simulink model "HW6_46"  (R2017a)
settings: Solver=VariableStepAuto  StartTime=0.0  StopTime=30  RelTol=1e-3
settings Model: Creator=USER  LastModifiedBy=dell

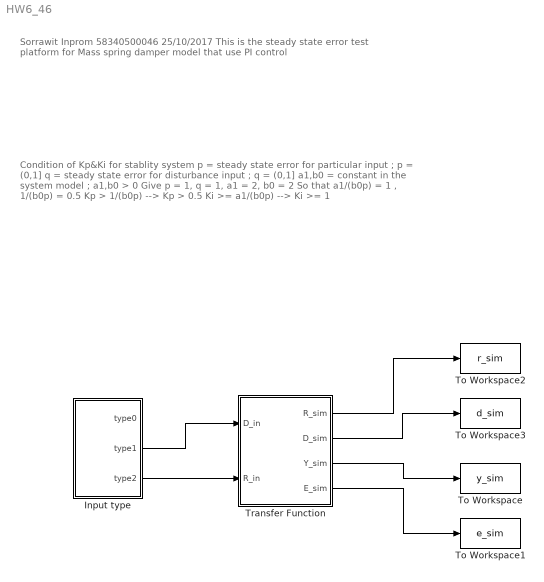
== system HW6_46 ==
  note: Sorrawit Inprom 58340500046
      | 25/10/2017
      |
      | This is the steady state error test platform
      | for Mass spring damper model that use PI control
  note: Condition of Kp&Ki for stablity system
      |
      | p = steady state error for particular input ; p = (0,1]
      | q = steady state error for disturbance input ; q = (0,1]
      | a1,b0 = constant in the system model ; a1,b0 > 0
      |
      | Give p = 1, q = 1, a1 = 2, b0 = 2
      |
      | So that a1/(b0p) = 1 , 1/(b0p) = 0.5
      |
      | Kp > 1/(b0p) --> Kp > 0.5
      | Ki >= a1/(b0p) --> Ki >= 1
  Input type : Subsystem
  To Workspace : ToWorkspace  VariableName=y_sim  SaveFormat=Timeseries  SampleTime=-1
  To Workspace1 : ToWorkspace  VariableName=e_sim  SaveFormat=Timeseries  SampleTime=-1
  To Workspace2 : ToWorkspace  VariableName=r_sim  SaveFormat=Timeseries  SampleTime=-1
  To Workspace3 : ToWorkspace  VariableName=d_sim  SaveFormat=Timeseries  SampleTime=-1
  Transfer Function : Subsystem  mask{a1=2, b0=2, Kp=1, Ki=1}
  wires:
  Transfer Function/1(R_sim) -> To Workspace2/1
  Transfer Function/2(D_sim) -> To Workspace3/1
  Transfer Function/3(Y_sim) -> To Workspace/1
  Transfer Function/4(E_sim) -> To Workspace1/1
  Input type/3(type2) -> Transfer Function/2(R_in)
  Input type/2(type1) -> Transfer Function/1(D_in)

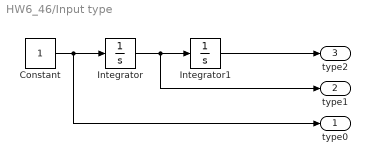
== system HW6_46/Input type ==
  Constant : Constant
  Integrator : Integrator
  Integrator1 : Integrator
  type0 : Outport
  type1 : Outport  Port=2
  type2 : Outport  Port=3
  wires:
  Integrator/1 -> type1/1, Integrator1/1
  Constant/1 -> type0/1, Integrator/1
  Integrator1/1 -> type2/1

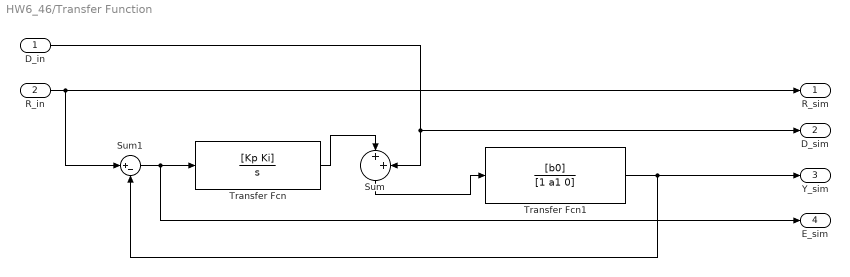
== system HW6_46/Transfer Function ==
  D_in : Inport
  R_in : Inport  Port=2
  Sum : Sum  Inputs=|++
  Sum1 : Sum  Inputs=|+-
  Transfer Fcn : TransferFcn  Numerator=[Kp Ki]  Denominator=[1 0]
  Transfer Fcn1 : TransferFcn  Numerator=[b0]  Denominator=[1 a1 0]
  R_sim : Outport
  D_sim : Outport  Port=2
  Y_sim : Outport  Port=3
  E_sim : Outport  Port=4
  wires:
  R_in/1 -> Sum1/1, R_sim/1
  Sum1/1 -> E_sim/1, Transfer Fcn/1
  Transfer Fcn/1 -> Sum/1
  Sum/1 -> Transfer Fcn1/1
  Transfer Fcn1/1 -> Sum1/2, Y_sim/1
  D_in/1 -> Sum/2, D_sim/1
